simulink model "can_test"  (R2020b)
settings: Solver=FixedStepDiscrete  StartTime=0.0  StopTime=10.0  FixedStep=0.01  RelTol=1e-3  EnableMultiTasking=on
InitFcn:
  | mbd_s32k_consistency_checks(bdroot(gcs));
undefined symbols (not defined in the file or in its folder): LQFP
libraries: mbd_s32k1xx_ec_toolbox x21, simulink x4
Description:
  | Sample code to demonstrate CAN Rx/Tx on CAN0 peripheral (500kb)
  | 
  | Extra Modules (In addition to template defaults):
  | None
  | 
  | For more information, see our Simulink CAN Guide:
  | https://www.audesseinc.com/labs/resources/can-guide/
  | 
  | Revision: 1.5
settings Model: LastModifiedBy=cbeal
settings DataIOCC: ExternalInput=off  InitialState=off  SaveOutput=off  SignalLogging=off  SaveTime=off
settings OptimizationCC: DefaultParameterBehavior=Inlined  DefaultUnderspecifiedDataType=single  OptimizeBlockIOStorage=off  EnhancedBackFolding=on  PassReuseOutputArgsAs=Individual arguments  OptimizeBlockOrder=speed  EfficientTunableParamExpr=on
settings DebuggingCC: InheritedTsInSrcMsg=none  SingleTaskRateTransMsg=error  ParameterTunabilityLossMsg=error  UnconnectedInputMsg=error  UnconnectedOutputMsg=error  UnconnectedLineMsg=error  UnknownTsInhSupMsg=error  ArithmeticOperatorsInVariantConditions=warning
settings HardwareCC: ProdBitPerPointer=32  ProdBitPerSizeT=32  ProdBitPerPtrDiffT=32  ProdLargestAtomicInteger=Long  ProdLargestAtomicFloat=Double  ProdWordSize=32  ProdHWDeviceType=ARM Compatible->ARM Cortex
settings SFSimCC: MATLABDynamicMemAlloc=off  CustomCodeUndefinedFunction=UseInterfaceOnly
settings RTWCC: Description=Model Based Design Toolbox S32K1xx Code Generation Target  SystemTargetFile=mbd_s32k.tlc  MakeCommand=mbd_s32k_make_rtw COPY_MDLREF_INCLUDES=0  TemplateMakefile=mbd_s32k.tmf  GenerateReport=on  IncludeHyperlinkInReport=on  LaunchReport=on  GenerateTraceInfo=on  GenerateTraceReport=on  GenerateTraceReportSl=on  GenerateTraceReportSf=on  GenerateTraceReportEml=on
settings CodeAppCC: ForceParamTrailComments=on  IgnoreCustomStorageClasses=off  OperatorAnnotations=on  SimulinkDataObjDesc=on  SFDataObjDesc=on  InsertBlockDesc=on  StateflowObjectComments=on
settings STFCustomTargetCC: TargetLangStandard=C99 (ISO)  MultiwordLength=256  ConcurrentExecutionCompliant=off  CombineOutputUpdateFcns=on  ERTCustomFileBanners=on  SupportContinuousTime=off  SupportNonInlinedSFcns=off  RemoveResetFunc=on  MATLABClassNameForMDSCustomization=Simulink.SoftwareTarget.ERTCustomization  CPPClassGenCompliant=off  GRTInterface=off  SystemTargetFile=mbd_s32k.tlc
settings ERTTargetCC: TargetLangStandard=C99 (ISO)  ParMdlRefBuildCompliant=off  CompOptLevelCompliant=off  ConcurrentExecutionCompliant=off  ModelStepFunctionPrototypeControlCompliant=off  CPPClassGenCompliant=off  UseToolchainInfoCompliant=off  InlinedParameterPlacement=NonHierarchical  ERTSrcFileBannerTemplate=mbd_ert_code_template.cgt  ERTHdrFileBannerTemplate=mbd_ert_code_template.cgt  ERTDataSrcFileTemplate=mbd_ert_code_template.cgt  ERTDataHdrFileTemplate=mbd_ert_code_template.cgt  ERTCustomFileTemplate=example_file_process.tlc

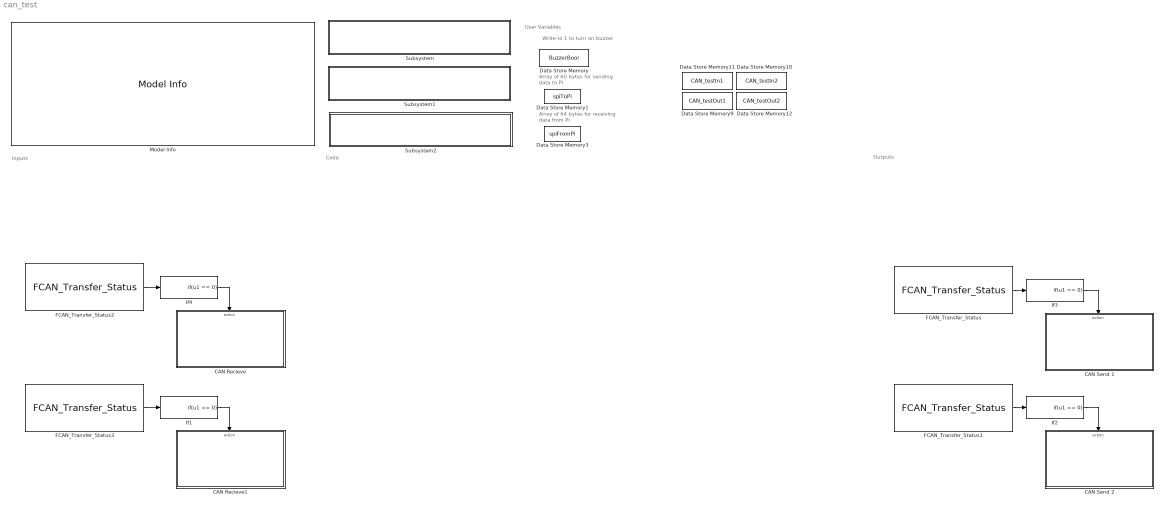
== system can_test ==
  note: User Variables
  note: Write to 1 to turn on buzzer
  note: Array of 60 bytes for sending data to Pi
  note: Inputs
  note: Code
  note: Outputs
  note: Array of 64 bytes for receiving data from Pi
  CAN Recieve : Subsystem  TreatAsAtomicUnit=on
  CAN Recieve1 : Subsystem  TreatAsAtomicUnit=on
  CAN Send 1 : Subsystem  TreatAsAtomicUnit=on
  CAN Send 2 : Subsystem  TreatAsAtomicUnit=on
  Data Store Memory : DataStoreMemory  DataStoreName=BuzzerBool  ReadBeforeWriteMsg=warning  WriteAfterWriteMsg=warning  WriteAfterReadMsg=warning  ShowAdditionalParam=off  OutDataTypeStr=boolean
  Data Store Memory1 : DataStoreMemory  DataStoreName=spiToPi  ReadBeforeWriteMsg=warning  WriteAfterWriteMsg=warning  WriteAfterReadMsg=warning  InitialValue=255*ones(1,60)  ShowAdditionalParam=off  OutDataTypeStr=uint8
  Data Store Memory10 : DataStoreMemory  DataStoreName=CAN_testIn2  ReadBeforeWriteMsg=warning  WriteAfterWriteMsg=warning  WriteAfterReadMsg=warning  ShowAdditionalParam=off  OutDataTypeStr=uint8  Dimensions=2
  Data Store Memory11 : DataStoreMemory  DataStoreName=CAN_testIn1  ReadBeforeWriteMsg=warning  WriteAfterWriteMsg=warning  WriteAfterReadMsg=warning  ShowAdditionalParam=off  OutDataTypeStr=uint8  Dimensions=8
  Data Store Memory12 : DataStoreMemory  DataStoreName=CAN_testOut2  ReadBeforeWriteMsg=warning  WriteAfterWriteMsg=warning  WriteAfterReadMsg=warning  ShowAdditionalParam=off  OutDataTypeStr=uint8
  Data Store Memory3 : DataStoreMemory  DataStoreName=spiFromPi  ReadBeforeWriteMsg=warning  WriteAfterWriteMsg=warning  WriteAfterReadMsg=warning  InitialValue=zeros(1,64)  ShowAdditionalParam=off  OutDataTypeStr=uint8
  Data Store Memory9 : DataStoreMemory  DataStoreName=CAN_testOut1  ReadBeforeWriteMsg=warning  WriteAfterWriteMsg=warning  WriteAfterReadMsg=warning  ShowAdditionalParam=off  OutDataTypeStr=uint8
  FCAN_Transfer_Status : mbd_s32k1xx_ec_toolbox/Communication Blocks/CAN Blocks/FCAN_Transfer_Status  can_instance=0  can_mb_idx=2
  FCAN_Transfer_Status1 : mbd_s32k1xx_ec_toolbox/Communication Blocks/CAN Blocks/FCAN_Transfer_Status  can_instance=0  can_mb_idx=3
  FCAN_Transfer_Status2 : mbd_s32k1xx_ec_toolbox/Communication Blocks/CAN Blocks/FCAN_Transfer_Status  can_instance=0  can_mb_idx=0
  FCAN_Transfer_Status3 : mbd_s32k1xx_ec_toolbox/Communication Blocks/CAN Blocks/FCAN_Transfer_Status  can_instance=0  can_mb_idx=1
  If{1..4} (4 alike) : If  IfExpression=u1 == 0  ShowElse=off
  Model Info : simulink/Model-Wide Utilities/Model Info  Frame=on  DisplayStringWithTags=|  HorizontalTextAlignment=Left  LeftAlignmentValue=0.02
      | Audesse Simulink Samples: %<ModelName>
      | 
      | %<Description>
  Subsystem : Subsystem  Priority=1
      mask Display:
      | scl=1/4;
      | patch(scl*[0,52,90,54],scl*[16,55,146,146],[16/255,118/255,188/255],'bottom-left');
      | patch(scl*[0,27,82,77,68],scl*[16,0,42,62,69],[46/255,49/255,146/255],'bottom-left');
      | patch(scl*[89,125,90,68],scl*[16,16,146,91],[0,0,0],'bottom-left');
      | disp('Hardware Modules Config\n(SPI,CAN,ADC,etc..)');
  Subsystem1 : Subsystem
      mask Display:
      | scl=1/4;
      | patch(scl*[0,52,90,54],scl*[16,55,146,146],[16/255,118/255,188/255],'bottom-left');
      | patch(scl*[0,27,82,77,68],scl*[16,0,42,62,69],[46/255,49/255,146/255],'bottom-left');
      | patch(scl*[89,125,90,68],scl*[16,16,146,91],[0,0,0],'bottom-left');
      | disp('Default Control Functions\n(Do not modify unless you know what you are doing)');
  Subsystem2 : Subsystem
      mask Display:
      | scl=1/4;
      | patch(scl*[0,52,90,54],scl*[16,55,146,146],[16/255,118/255,188/255],'bottom-left');
      | patch(scl*[0,27,82,77,68],scl*[16,0,42,62,69],[46/255,49/255,146/255],'bottom-left');
      | patch(scl*[89,125,90,68],scl*[16,16,146,91],[0,0,0],'bottom-left');
      | disp('Run Once at Startup');
  wires:
  FCAN_Transfer_Status3/1 -> If1/1
  If1/1 -> CAN Recieve1/Action
  FCAN_Transfer_Status2/1 -> If4/1
  If4/1 -> CAN Recieve/Action
  FCAN_Transfer_Status/1 -> If3/1
  If2/1 -> CAN Send 2/Action
  FCAN_Transfer_Status1/1 -> If2/1
  If3/1 -> CAN Send 1/Action

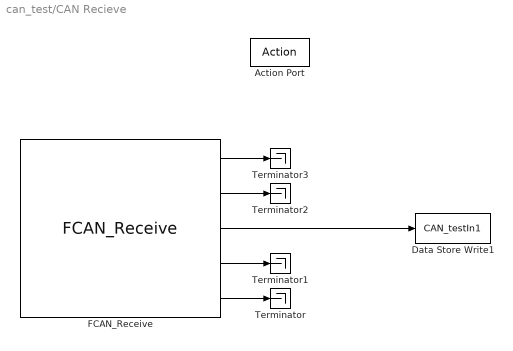
== system can_test/CAN Recieve ==
  Action Port : ActionPort  ActionPortLabel=if(u1 == 0)
  Data Store Write1 : DataStoreWrite  DataStoreName=CAN_testIn1
  FCAN_Receive : mbd_s32k1xx_ec_toolbox/Communication Blocks/CAN Blocks/FCAN_Receive  can_instance=0  can_mode=Blocking  can_timeout_ms=2  can_mb_idx=0  can_extended_id=off  can_is_remote=off  can_id=58b  can_msg_mask=FFFFFFFF  show_adv_opts=off  can_use_rxfifo=off  can_fd_enable=off
  Terminator{,1..3} (4 alike) : Terminator
  wires:
  FCAN_Receive/2 -> Terminator2/1
  FCAN_Receive/4 -> Terminator1/1
  FCAN_Receive/5 -> Terminator/1
  FCAN_Receive/1 -> Terminator3/1
  FCAN_Receive/3 -> Data Store Write1/1

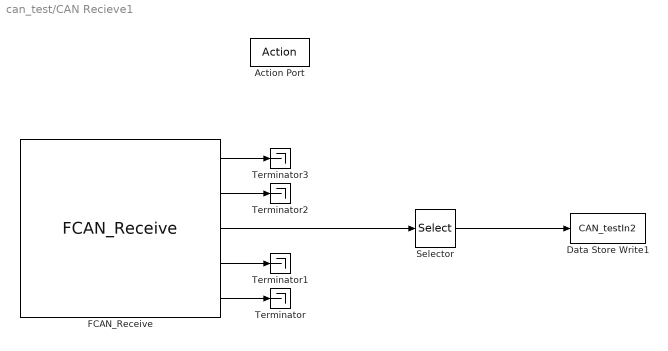
== system can_test/CAN Recieve1 ==
  Action Port : ActionPort  ActionPortLabel=if(u1 == 0)
  Data Store Write1 : DataStoreWrite  DataStoreName=CAN_testIn2
  FCAN_Receive : mbd_s32k1xx_ec_toolbox/Communication Blocks/CAN Blocks/FCAN_Receive  can_instance=0  can_mode=Blocking  can_timeout_ms=2  can_mb_idx=1  can_extended_id=off  can_is_remote=off  can_id=18b  can_msg_mask=FFFFFFFF  show_adv_opts=off  can_use_rxfifo=off  can_fd_enable=off
  Selector : Selector  InputPortWidth=8  IndexOptions=Index vector (dialog)  Indices=[1 2]  OutputSizes=1
  Terminator{,1..3} (4 alike) : Terminator
  wires:
  FCAN_Receive/2 -> Terminator2/1
  Selector/1 -> Data Store Write1/1
  FCAN_Receive/4 -> Terminator1/1
  FCAN_Receive/5 -> Terminator/1
  FCAN_Receive/1 -> Terminator3/1
  FCAN_Receive/3 -> Selector/1

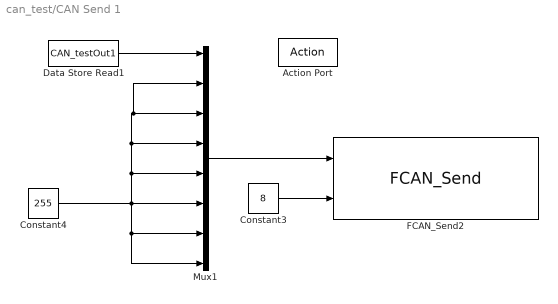
== system can_test/CAN Send 1 ==
  Action Port : ActionPort  ActionPortLabel=if(u1 == 0)
  Constant3 : Constant  Value=8  OutDataTypeStr=uint8
  Constant4 : Constant  Value=255  OutDataTypeStr=uint8
  Data Store Read1 : DataStoreRead  DataStoreName=CAN_testOut1
  FCAN_Send2 : mbd_s32k1xx_ec_toolbox/Communication Blocks/CAN Blocks/FCAN_Send  can_instance=0  can_mode=Non-blocking  can_timeout_ms=0  can_mb_idx=2  can_extended_id=off  can_is_remote=off  can_id=333  show_adv_opts=off  can_fd_enable=off  can_enable_brs=off  can_fd_padding=0
  Mux1 : Mux  Inputs=8
  wires:
  Mux1/1 -> FCAN_Send2/1
  Data Store Read1/1 -> Mux1/1
  Constant3/1 -> FCAN_Send2/2
  Constant4/1 -> Mux1/8, Mux1/7, Mux1/6, Mux1/2, Mux1/3, Mux1/4, Mux1/5

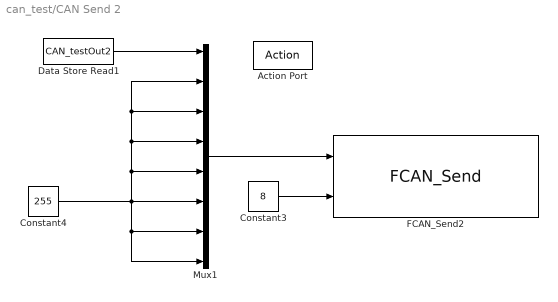
== system can_test/CAN Send 2 ==
  Action Port : ActionPort  ActionPortLabel=if(u1 == 0)
  Constant3 : Constant  Value=8  OutDataTypeStr=uint8
  Constant4 : Constant  Value=255  OutDataTypeStr=uint8
  Data Store Read1 : DataStoreRead  DataStoreName=CAN_testOut2
  FCAN_Send2 : mbd_s32k1xx_ec_toolbox/Communication Blocks/CAN Blocks/FCAN_Send  can_instance=0  can_mode=Non-blocking  can_timeout_ms=0  can_mb_idx=3  can_extended_id=off  can_is_remote=off  can_id=444  show_adv_opts=off  can_fd_enable=off  can_enable_brs=off  can_fd_padding=0
  Mux1 : Mux  Inputs=8
  wires:
  Mux1/1 -> FCAN_Send2/1
  Data Store Read1/1 -> Mux1/1
  Constant3/1 -> FCAN_Send2/2
  Constant4/1 -> Mux1/8, Mux1/7, Mux1/6, Mux1/2, Mux1/3, Mux1/4, Mux1/5

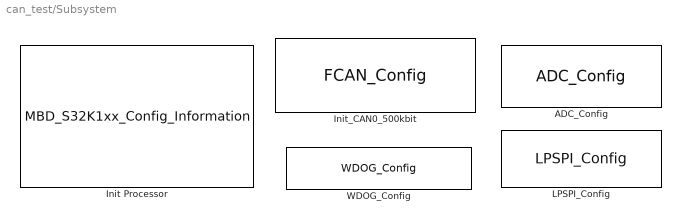
== system can_test/Subsystem ==
  ADC_Config : mbd_s32k1xx_ec_toolbox/Motor Control Blocks/ADC Blocks/ADC_Config  instance=0  mode=12-bit conversion  smplts=20  adiclk=alternate clock 1  adiv=input clock  show_adv_opts=on  pretrgsel=PDB pre-trigger  swpretrg=Disabled  adtrg=software  trgsel=TRGMUX output  refsel=Vrefh and Vrefl  supply_monitoring=off  acfe=off  acfgt=off  acren=off  cv1=0  cv2=0  adco=off  avge=off  avgs=4 samples
  Init Processor : mbd_s32k1xx_ec_toolbox/MBD_S32K1xx_Config_Information  mbdt_ver=0  disp_str=|  config_params=[]  mcu_target_name=S32K144  mcu_target_package=100-LQFP  mcu_target_sram_size=64KB  mcu_system_clock_freq=80  mcu_xtal_freq=External 8  mcu_steptick_timer=LPIT Channel 0  mcu_steptick_prio=15  ds_import_enable=on  target_compiler=GCC  target_memory=FLASH  gcc_target_compile_opts=-mcpu=cortex-m4 -mthumb -mfloat-abi=hard -mfpu=fpv4-sp-d16 -O1 -g -gstrict-dwarf  gcc_target_assemble_opts=-mcpu=cortex-m4 -mthumb -mfloat-abi=hard -mfpu=fpv4-sp-d16 -g  gcc_target_link_opts=-mcpu=cortex-m4 -mthumb -mfloat-abi=hard -mfpu=fpv4-sp-d16  gcc_target_default_lcf=on  gcc_target_user_lcf=S32K148_192_flash.ld  ghs_target_compile_opts=-cpu=cortexm4f -thumb -DARM_MATH_CM4 -fpu=vfpv4_d16 -fsingle -Ogeneral -Wundef -Wimplicit-int -Wshadow -Wtrigraphs --no_commons --gnu_asm -gnu99 -gdwarf-2 -G  ghs_target_assemble_opts=-cpu=cortexm4f -fpu=vfpv4_d16  ghs_target_link_opts=-cpu=cortexm4f -thumb -fpu=vfpv4_d16  ghs_target_default_lcf=on  ghs_target_user_lcf=S32K148_192_flash.ld  iar_target_compile_opts=--cpu=Cortex-M4F --thumb --fpu=VFPv4_sp -Ol -e --debug --dlib_config normal  iar_target_assemble_opts=--cpu Cortex-M4F --thumb --fpu VFPv4_sp  iar_target_link_opts=--no_exceptions --vfe --inline  iar_target_default_lcf=on  iar_target_user_lcf=S32K148_192_flash.icf  pil_download_enable=off  rbl_download_enable=off  rbl_start_delay=5000000  rbl_download_interface=OpenSDA  rbl_restart_request=off  rbl_com_port=Custom  rbl_com_port_custom=COM1  pil_download_rate=57600  pil_opensda_drive=Custom  pil_opensda_drive_custom=D  pil_uart_instance=1  pil_uart_rx=PTC6: [LPUART1_RX | Receive]  pil_uart_tx=PTC7: [LPUART1_TX | Transmit]  FTM_PWM_PcrCheckEnDis=on  FTM_Input_Edge_Inputs_PcrCheckEnDis=on  FTM_Dual_Edge_Inputs_PcrCheckEnDis=on  FTM_Quadrature_Inputs_PcrCheckEnDis=on  FTM_Hall_Sensor_Inputs_PcrCheckEnDis=on  LPTMR_PcrCheckEnDis=on  PIT_PcrCheckEnDis=on  RTC_PcrCheckEnDis=on  FlexCAN_PcrCheckEnDis=on  LIN_PcrCheckEnDis=on  FlexIO_PcrCheckEnDis=on  LPI2C_PcrCheckEnDis=on  LPSPI_PcrCheckEnDis=on  LPUART_PcrCheckEnDis=on  CMP_PcrCheckEnDis=on  GPIO_OutputPcrCheckEnDis=on  GPIO_InputPcrCheckEnDis=on  SBC_PcrCheckEnDis=on  BMS_PcrCheckEnDis=on  AMMCLIB_PcrCheckEnDis=on  FM_PcrCheckEnDis=on  Profile_PcrCheckEnDis=on  ConfigParams_PcrCheckEnDis=on  ModelRef_PcrCheckEnDis=on  PDB0_PcrCheckEnDis=on  CSEc_PcrCheckEnDis=on  eDMA_PcrCheckEnDis=on  FLASH_PcrCheckEnDis=on  ADC_PcrCheckEnDis=on  WDOG_PcrCheckEnDis=on
      | Target : S32K144-64KB_SRAM
      | Package : 100-pin
      | System clock : 80 MHz
      | XTAL clock : External 8 MHz
      | Compiler : IAR
      | Target Type : FLASH
      | Download Code after build : off
      | Step Tick Interrupt Priority : 15
  Init_CAN0_500kbit : mbd_s32k1xx_ec_toolbox/Communication Blocks/CAN Blocks/FCAN_Config  can_instance=0  can_mode=Normal mode  can_max_num_mb=16  can_rx=PTB0: [CAN0_RX | CAN Rx channel]  can_tx=PTB1: [CAN0_TX | CAN Tx Channel]  show_adv_opts=off  can_clk_src=Peripheral clock  bitrate=500  bitrate_adv_opts=off  can_presdiv=7  can_rjw=3  can_pseg1=6  can_pseg2=3  can_propseg=7  can_cbt_presdiv=9  can_cbt_rjw=0  can_cbt_pseg1=3  can_cbt_pseg2=3  can_cbt_propseg=6  can_fd_enable=off  can_payload=8  can_rxfifo_enable=off  can_fifo_id_filter_extended=off  can_fifo_id_filter_remote=off  can_num_id_filters=8  can_fifo_id_format=A  can_fifo_id_filter={'0x0', '0x0', '0x0', '0x0', '0x0', '0x0', '0x0', '0x0'}  can_pn_enable=off  can_wakeup_match=off  can_wakeup_timeout=off  can_timeout_en=off  can_match_timeout=1  can_multiple_matches_en=off  can_num_matches=1  can_idfilter_extendedid=off  can_idfilter_remoteframe=off  can_idfilter_type=Match exact  can_idfilter_id1=0  can_idfilter_id2=0  can_payloadfilter_enable=on  can_payloadfilter_dlclow=0  can_payloadfilter_dlchigh=0  can_payloadfilter_type=Match exact  can_payloadfilter_payload1_b0=0  can_payloadfilter_payload1_b1=0  can_payloadfilter_payload1_b2=0  can_payloadfilter_payload1_b3=0  can_payloadfilter_payload1_b4=0  can_payloadfilter_payload1_b5=0  can_payloadfilter_payload1_b6=0  can_payloadfilter_payload1_b7=0  can_payloadfilter_payload2_b0=0  can_payloadfilter_payload2_b1=0  can_payloadfilter_payload2_b2=0  can_payloadfilter_payload2_b3=0  can_payloadfilter_payload2_b4=0  can_payloadfilter_payload2_b5=0  can_payloadfilter_payload2_b6=0  can_payloadfilter_payload2_b7=0
  "LPSPI_Config " : mbd_s32k1xx_ec_toolbox/Communication Blocks/SPI Blocks/LPSPI_Config   InstanceNumber=1  Role=Slave  BaudRate=10000  ShowAdvanced=on  sin=PTB15: [LPSPI1_SIN | LPSPI Serial Data Input]  sout=PTB16: [LPSPI1_SOUT | LPSPI Serial Data Output]  sck=PTB14: [LPSPI1_SCK | LPSPI Serial Clock I/O]  pcs0=None  pcs1=None  pcs2=None  pcs3=PTB17: [LPSPI1_PCS3 | Peripheral Chip Select 3]  CPHA=1  CPOL=0  BitOrder=MSB first  TransferSize=8  WhichPCS=0  PCSPol=ActiveLow  ContinuousTransfer=on
  WDOG_Config : mbd_s32k1xx_ec_toolbox/Core and System Blocks/WDOG Blocks/WDOG_Config  clk_source=LPO clock  window_enable=off  window_value=1000.000 milliseconds  timeout_value=1000.000 milliseconds  prescaler_enable=on  update_enable=off  int_enable=off  show_adv_opts=on

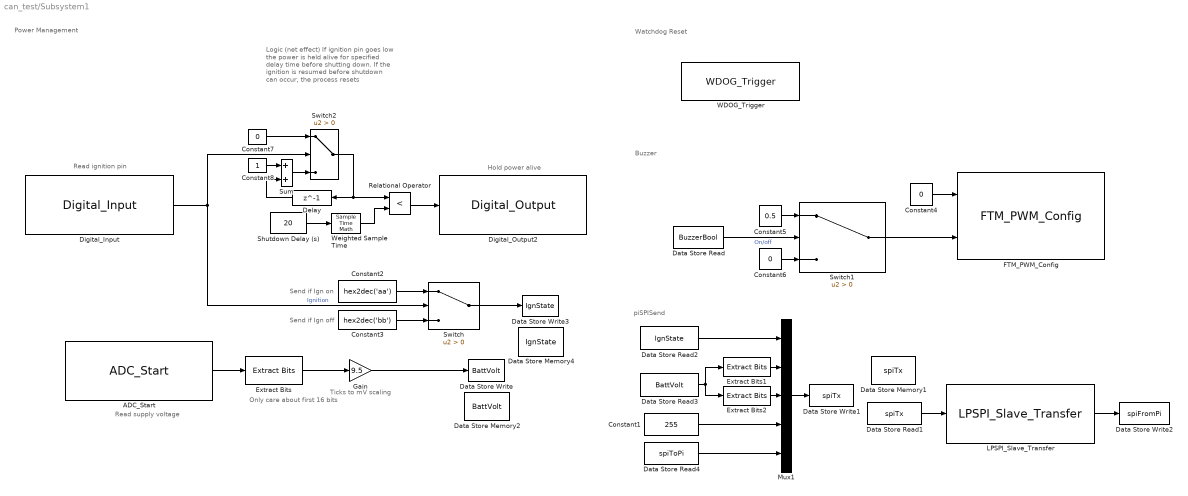
== system can_test/Subsystem1 ==
  note: piSPISend
  note: Watchdog Reset
  note: Power Management
  note: Read ignition pin
  note: Only care about
      | first 16 bits
  note: Ticks to mV scaling
  note: Read supply voltage
  note: Send if Ign on
  note: Send if Ign off
  note: Buzzer
  note: Logic (net effect)
      | If ignition pin goes low the power is held alive for specified delay time before shutting down.
      |
      | If the ignition is resumed before shutdown can occur, the process resets
  note: Hold power alive
  ADC_Start : mbd_s32k1xx_ec_toolbox/Motor Control Blocks/ADC Blocks/ADC_Start  instance=0  adc_r=A  adc_chan=PTA6: [ADC0_SE2 | ADC Single Ended Input]  aien=off  mcuTargetUpdate=on
  Constant1 : Constant  Value=255  OutDataTypeStr=uint8
  Constant2 : Constant  Value=hex2dec('aa')  OutDataTypeStr=uint8
  Constant3 : Constant  Value=hex2dec('bb')  OutDataTypeStr=uint8
  Constant4 : Constant  Value=0  OutDataTypeStr=single
  Constant5 : Constant  Value=0.5  OutDataTypeStr=single
  Constant6 : Constant  Value=0  OutDataTypeStr=single
  Constant7 : Constant  Value=0  OutDataTypeStr=uint8
  Constant8 : Constant  OutDataTypeStr=uint8
  Data Store Memory1 : DataStoreMemory  DataStoreName=spiTx  ReadBeforeWriteMsg=warning  WriteAfterWriteMsg=warning  WriteAfterReadMsg=warning  InitialValue=zeros(1,64)  ShowAdditionalParam=off  OutDataTypeStr=uint8
  Data Store Memory2 : DataStoreMemory  DataStoreName=BattVolt  ReadBeforeWriteMsg=warning  WriteAfterWriteMsg=warning  WriteAfterReadMsg=warning  InitialValue=[0]  ShowAdditionalParam=off  OutDataTypeStr=uint16
  Data Store Memory4 : DataStoreMemory  DataStoreName=IgnState  ReadBeforeWriteMsg=warning  WriteAfterWriteMsg=warning  WriteAfterReadMsg=warning  InitialValue=[170]  ShowAdditionalParam=off  OutDataTypeStr=uint8
  Data Store Read : DataStoreRead  DataStoreName=BuzzerBool
  Data Store Read1 : DataStoreRead  DataStoreName=spiTx
  Data Store Read2 : DataStoreRead  DataStoreName=IgnState
  Data Store Read3 : DataStoreRead  DataStoreName=BattVolt
  Data Store Read4 : DataStoreRead  DataStoreName=spiToPi
  Data Store Write : DataStoreWrite  DataStoreName=BattVolt
  Data Store Write1 : DataStoreWrite  DataStoreName=spiTx
  Data Store Write2 : DataStoreWrite  DataStoreName=spiFromPi
  Data Store Write3 : DataStoreWrite  DataStoreName=IgnState
  Delay : Delay  DelayLength=1  InitialCondition=0
  Digital_Input : mbd_s32k1xx_ec_toolbox/GPIO Blocks/Digital_Input  gpio_pin=PTE13: [PTE13 | Port E I/O]  pull_resistor=Pulldown  passive_filter=off
  Digital_Output2 : mbd_s32k1xx_ec_toolbox/GPIO Blocks/Digital_Output  gpio_pin=PTD7: [PTD7 | Port D I/O]  init_val=High  drive_strength=Low
  Extract Bits : simulink/Logic and Bit Operations/Extract Bits  bitsToExtract=Lower half  numBits=8  bitIdxRange=[0 7]  outScalingMode=Treat bit field as an integer
  Extract Bits1 : simulink/Logic and Bit Operations/Extract Bits  bitsToExtract=Upper half  numBits=8  bitIdxRange=[0 7]  outScalingMode=Treat bit field as an integer
  Extract Bits2 : simulink/Logic and Bit Operations/Extract Bits  bitsToExtract=Lower half  numBits=8  bitIdxRange=[0 7]  outScalingMode=Treat bit field as an integer
  FTM_PWM_Config : mbd_s32k1xx_ec_toolbox/Motor Control Blocks/FTM Blocks/FTM_PWM_Config  ftmModule=2  ftmMode=Edge-Aligned PWM  ftmSourceClock=80 MHz  swcontrol_enable=off  chan0En=off  chan0Type=Complementary  chan2En=on  chan2Type=Independent  chan4En=off  chan4Type=Independent  chan6En=off  chan6Type=Independent  ftmPwmUnits=Hz  outFrequency=4000  ftmPeriod=20000  ftmPrescaler=Divide by 1  deadtimeUnits=Nanoseconds  deadtimeNs=0  deadtimeTicks=0  deadtimePrescaler=Divide by 1  dutyCycleCh0=0.25  dutyCycleCh1=0.25  dutyCycleCh2=0  dutyCycleCh3=0.5  dutyCycleCh4=0.25  dutyCycleCh5=0.25  dutyCycleCh6=0.25  dutyCycleCh7=0.25  dutyCycleSim=off  startAfterInit=on  showAdvOpt=on  pinFtmCh0=PTC5: [FTM2_CH0 | FTM Channel]  pinFtmCh1=None  pinPolCh0=Active Low  pinPolCh1=Active Low  outputComplem0=Main duplicated  outputLevel0=Low  outputLevel1=Low  pinFtmCh2=PTE4: [FTM2_CH2 | FTM Channel]  pinFtmCh3=PTD5: [FTM2_CH3 | FTM Channel]  pinPolCh2=Active Low  pinPolCh3=Active High  outputComplem2=Main duplicated  outputLevel2=High  outputLevel3=Low  pinFtmCh4=PTD13: [FTM2_CH4 | FTM Channel]  pinFtmCh5=None  pinPolCh4=Active Low  pinPolCh5=Active Low  outputComplem4=Main duplicated  outputLevel4=Low  outputLevel5=Low  pinFtmCh6=PTC12: [FTM2_CH6 | FTM Channel]  pinFtmCh7=None  pinPolCh6=Active Low  pinPolCh7=Active Low  outputComplem6=Main duplicated  outputLevel6=Low  outputLevel7=Low  initTrigger=off  chTrigger0=off  chTrigger1=off  chTrigger2=off  chTrigger3=off  chTrigger4=off  chTrigger5=off  chTrigger6=off  chTrigger7=off  mcuTargetUpdate=on  pwmSyncTrg=Software trigger  pwmSyncHwRouting=TRGMUX_FTM7  pwmSyncTrg0=off  pwmSyncTrg1=off  pwmSyncTrg2=off  pwmSyncAutoClear=on  pwmSyncMinLoad=on  pwmSyncMaxLoad=on  pwmSyncInvert=System Clock  pwmSyncOutControl=System Clock  pwmSyncOutMask=System Clock  pwmSyncCounterInitial=System Clock  pwmSyncPoints=Update now  reloadEnable=off  reloadPriority=15  reloadHalfCycle=off  reloadHCR=0  reloadFrequency=0  chnMatch0=off  chnMatch1=off  chnMatch2=off  chnMatch3=off  chnMatch4=off  chnMatch5=off  chnMatch6=off  chnMatch7=off  pwmFaultProtection=off  pwmFaultInterrupt=off  pwmFaultClearing=Fault control disabled  pwmFaultPinState=Safe Value  pwmFaultFilterValue=0  pwmFaultPriority=15  fault_disen_0=off  fault_filter_0=off  fault_polarity_0=Active High  fault_disen_1=off  fault_filter_1=off  fault_polarity_1=Active high  fault_disen_2=off  fault_filter_2=off  fault_polarity_2=Active high  fault_disen_3=off  fault_filter_3=off  fault_polarity_3=Active high  fault_pin_0=None  fault_pin_1=None  fault_pin_2=None  fault_pin_3=None
  Gain : Gain  Gain=9.5  OutDataTypeStr=uint16
  LPSPI_Slave_Transfer : mbd_s32k1xx_ec_toolbox/Communication Blocks/SPI Blocks/LPSPI_Slave_Transfer  instance=1  pcs=3  pcs_polarity=ActiveLow  xfermode=Non blocking  timeout=70  spi_upd=on
  Mux1 : Mux  Inputs=5
  Relational Operator : RelationalOperator  Operator=<  OutDataTypeStr=boolean  RndMeth=Simplest  InputSameDT=on
  Shutdown Delay (s) : Constant  Value=20  OutDataTypeStr=uint32
  Sum : Sum
  Switch : Switch  Criteria=u2 > Threshold
  Switch1 : Switch  Criteria=u2 > Threshold  OutDataTypeStr=single
  Switch2 : Switch  Criteria=u2 > Threshold  OutDataTypeStr=uint32
  WDOG_Trigger : mbd_s32k1xx_ec_toolbox/Core and System Blocks/WDOG Blocks/WDOG_Trigger
  Weighted Sample Time : SampleTimeMath  TsampMathOp=/  OutDataTypeStr=Inherit: Inherit via back propagation  RndMeth=Round  SaturateOnIntegerOverflow=on
  wires:
  Constant3/1 -> Switch/3
  Constant2/1 -> Switch/1
  Extract Bits/1 -> Gain/1
  ADC_Start/1 -> Extract Bits/1
  Switch/1 -> Data Store Write3/1
  Data Store Read/1 -> Switch1/2  "On/off"
  Switch1/1 -> FTM_PWM_Config/2
  Constant5/1 -> Switch1/1
  Constant4/1 -> FTM_PWM_Config/1
  Constant6/1 -> Switch1/3
  Data Store Read2/1 -> Mux1/1
  Mux1/1 -> Data Store Write1/1
  Data Store Read1/1 -> LPSPI_Slave_Transfer/1
  LPSPI_Slave_Transfer/1 -> Data Store Write2/1
  Gain/1 -> Data Store Write/1
  Constant1/1 -> Mux1/4
  Data Store Read4/1 -> Mux1/5
  Extract Bits2/1 -> Mux1/3
  Extract Bits1/1 -> Mux1/2
  Data Store Read3/1 -> Extract Bits2/1, Extract Bits1/1
  Switch2/1 -> Delay/1, Relational Operator/1
  Weighted Sample Time/1 -> Relational Operator/2
  Relational Operator/1 -> Digital_Output2/1
  Shutdown Delay (s)/1 -> Weighted Sample Time/1
  Constant7/1 -> Switch2/1
  Sum/1 -> Switch2/3
  Constant8/1 -> Sum/1
  Delay/1 -> Sum/2
  Digital_Input/1 -> Switch2/2, Switch/2  "Ignition"

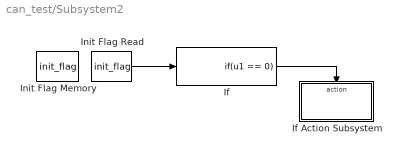
== system can_test/Subsystem2 ==
  If : If  IfExpression=u1 == 0  ShowElse=off
  If Action Subsystem : Subsystem  TreatAsAtomicUnit=on
  Init Flag Memory : DataStoreMemory  DataStoreName=init_flag  ReadBeforeWriteMsg=warning  WriteAfterWriteMsg=warning  WriteAfterReadMsg=warning  ShowAdditionalParam=off  OutDataTypeStr=uint32
  Init Flag Read : DataStoreRead  DataStoreName=init_flag
  wires:
  Init Flag Read/1 -> If/1
  If/1 -> If Action Subsystem/Action

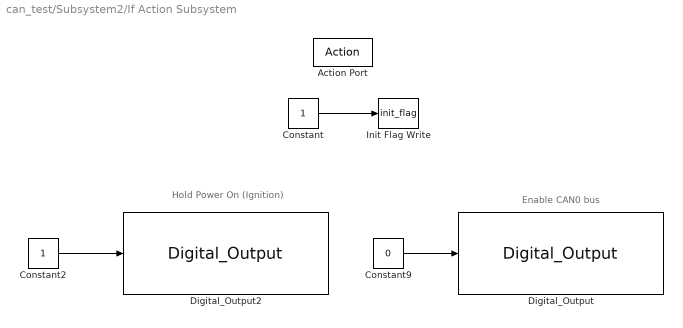
== system can_test/Subsystem2/If Action Subsystem ==
  note: Enable CAN0 bus
  note: Hold Power On (Ignition)
  Action Port : ActionPort  ActionPortLabel=if(u1 == 0)
  Constant : Constant  OutDataTypeStr=uint32
  Constant2 : Constant  OutDataTypeStr=Inherit: Inherit via back propagation
  Constant9 : Constant  Value=0  OutDataTypeStr=Inherit: Inherit via back propagation
  Digital_Output : mbd_s32k1xx_ec_toolbox/GPIO Blocks/Digital_Output  gpio_pin=PTC10: [PTC10 | Port C I/O]  init_val=Low  drive_strength=Low
  Digital_Output2 : mbd_s32k1xx_ec_toolbox/GPIO Blocks/Digital_Output  gpio_pin=PTD7: [PTD7 | Port D I/O]  init_val=High  drive_strength=Low
  Init Flag Write : DataStoreWrite  DataStoreName=init_flag
  wires:
  Constant/1 -> Init Flag Write/1
  Constant9/1 -> Digital_Output/1
  Constant2/1 -> Digital_Output2/1
